simulink model "PID_C_R_Simulink_1_0_OLC"  (R2020a)
settings: Solver=FixedStepAuto  StartTime=0.0  StopTime=inf  RelTol=1e-3  EnableMultiTasking=on
libraries: arduinolib x8, simulink x2
Description:
  | __Simple PID driven robot
  | ___Open loop control
settings Model: SILPILModeSetting=veronly  ExtModeTrigDuration=2  Creator=Mohanad M.Marzouk  LastModifiedBy=Mohanad M.Marzouk
settings SolverCC: AutoInsertRateTranBlk=on
settings OptimizationCC: EnhancedBackFolding=on  PassReuseOutputArgsAs=Individual arguments  ZeroExternalMemoryAtStartup=off  ZeroInternalMemoryAtStartup=off  MaxStackSize=64  OptimizeBlockOrder=speed  DifferentSizesBufferReuse=on  OptimizationCustomize=off  EfficientTunableParamExpr=on
settings DebuggingCC: ParameterTunabilityLossMsg=error
settings HardwareCC: ProdBitPerInt=16  ProdBitPerPointer=16  ProdBitPerSizeT=16  ProdBitPerPtrDiffT=16  ProdLargestAtomicFloat=None  ProdWordSize=8  ProdHWDeviceType=Atmel->AVR
settings SFSimCC: MATLABDynamicMemAlloc=off
settings RTWCC: SystemTargetFile=ert.tlc  HardwareBoard=Arduino Mega 2560  TLCOptions=-aInlineSetEventsForThisBaseRateFcn=TLC_FALSE -aSuppressMultiTaskScheduler=TLC_FALSE -aRateBasedStepFcn=1  GenCodeOnly=on  TemplateMakefile=ert_default_tmf  Toolchain=Arduino AVR  BuildConfiguration=Faster Runs
settings CodeAppCC: ForceParamTrailComments=on  IgnoreCustomStorageClasses=off  OperatorAnnotations=on  SimulinkDataObjDesc=on  SFDataObjDesc=on  InsertBlockDesc=on
settings ERTTargetCC: SupportContinuousTime=on  SupportVariableSizeSignals=on  ExtModeStaticAllocSize=2048

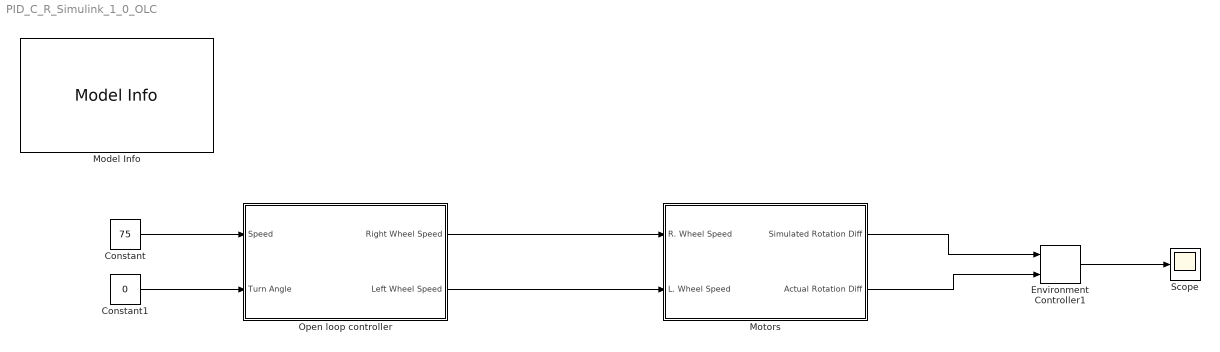
== system PID_C_R_Simulink_1_0_OLC ==
  Constant : Constant  Value=75
  Constant1 : Constant  Value=0
  Environment Controller1 : simulink/Signal Routing/Environment Controller
      settings: SourceProductBaseCode=SL
  Model Info : simulink/Model-Wide Utilities/Model Info  Frame=on  DisplayStringWithTags=|  HorizontalTextAlignment=Left  LeftAlignmentValue=0.02
      | Model Info
      | ---------------------------------------------
      | %<Created>
      | %<Creator>
      | %<ModelVersion>
      | %<ModelName>
      | %<Description>
      | %<LastModifiedBy>
      | %<LastModificationDate>
  Motors : Subsystem
  Open loop controller : Subsystem
  Scope : Scope
  wires:
  Environment Controller1/1 -> Scope/1
  Constant/1 -> Open loop controller/1(Speed)
  Constant1/1 -> Open loop controller/2(Turn Angle)
  Motors/1(Simulated Rotation Diff) -> Environment Controller1/1
  Motors/2(Actual Rotation Diff) -> Environment Controller1/2
  Open loop controller/1(Right Wheel Speed) -> Motors/1(R. Wheel Speed)
  Open loop controller/2(Left Wheel Speed) -> Motors/2(L. Wheel Speed)

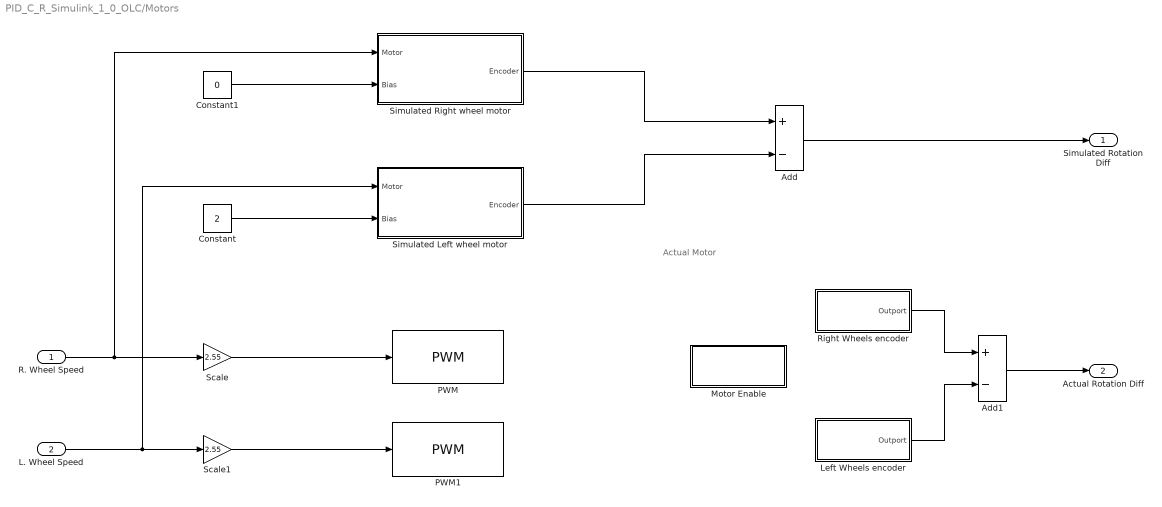
== system PID_C_R_Simulink_1_0_OLC/Motors ==
  note: Actual Motor
  R. Wheel Speed : Inport
  L. Wheel Speed : Inport  Port=2
  Add : Sum  Inputs=+-
  Add1 : Sum  Inputs=+-
  Constant : Constant  Value=2
  Constant1 : Constant  Value=0
  Left Wheels encoder : Subsystem
  Motor Enable : Subsystem
  PWM : arduinolib/PWM  pinNumber=10  frequencyType=Default  desiredFrequency=490.2  achievableFrequency=490.2
  PWM1 : arduinolib/PWM  pinNumber=11  frequencyType=Default  desiredFrequency=490.2  achievableFrequency=490.2
  Right Wheels encoder : Subsystem
  Scale : Gain  Gain=2.55
  Scale1 : Gain  Gain=2.55
  Simulated Left wheel motor : Subsystem
  Simulated Right wheel motor : Subsystem
  Simulated Rotation Diff : Outport
  Actual Rotation Diff : Outport  Port=2
  wires:
  Scale/1 -> PWM/1
  Scale1/1 -> PWM1/1
  L. Wheel Speed/1 -> Simulated Left wheel motor/1(Motor), Scale1/1
  R. Wheel Speed/1 -> Simulated Right wheel motor/1(Motor), Scale/1
  Constant/1 -> Simulated Left wheel motor/2(Bias)
  Constant1/1 -> Simulated Right wheel motor/2(Bias)
  Simulated Right wheel motor/1(Encoder) -> Add/1
  Simulated Left wheel motor/1(Encoder) -> Add/2
  Add/1 -> Simulated Rotation Diff/1
  Add1/1 -> Actual Rotation Diff/1
  Left Wheels encoder/1(Outport) -> Add1/2
  Right Wheels encoder/1(Outport) -> Add1/1

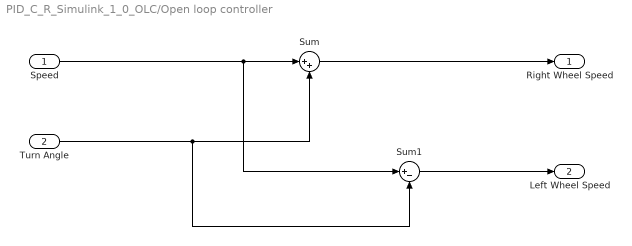
== system PID_C_R_Simulink_1_0_OLC/Open loop controller ==
  Speed : Inport
  Turn Angle : Inport  Port=2
  Sum : Sum  Inputs=|++
  Sum1 : Sum  Inputs=|+-
  Right Wheel Speed : Outport
  Left Wheel Speed : Outport  Port=2
  wires:
  Sum/1 -> Right Wheel Speed/1
  Sum1/1 -> Left Wheel Speed/1
  Turn Angle/1 -> Sum1/2, Sum/2
  Speed/1 -> Sum1/1, Sum/1

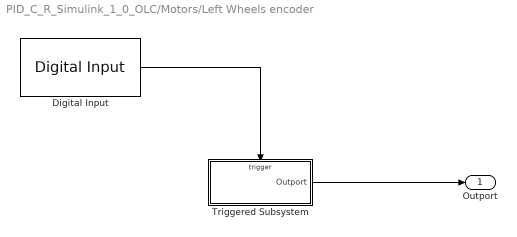
== system PID_C_R_Simulink_1_0_OLC/Motors/Left Wheels encoder ==
  Digital Input : arduinolib/Digital Input  pinNumber=9  Direction=input  SampleTime=0.001  blockPlatform=arduino
  Triggered Subsystem : Subsystem  TreatAsAtomicUnit=on
  Outport : Outport
  wires:
  Digital Input/1 -> Triggered Subsystem/Trigger
  Triggered Subsystem/1(Outport) -> Outport/1

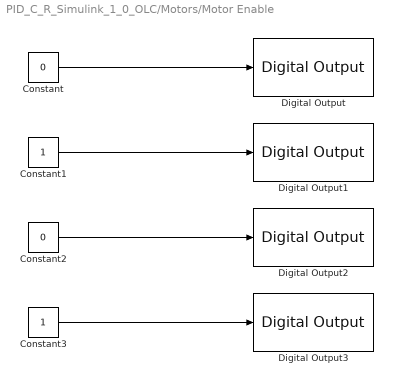
== system PID_C_R_Simulink_1_0_OLC/Motors/Motor Enable ==
  Constant : Constant  Value=0
  Constant1 : Constant
  Constant2 : Constant  Value=0
  Constant3 : Constant
  Digital Output : arduinolib/Digital Output  pinNumber=4  Direction=output  blockPlatform=arduino
  Digital Output1 : arduinolib/Digital Output  pinNumber=5  Direction=output  blockPlatform=arduino
  Digital Output2 : arduinolib/Digital Output  pinNumber=2  Direction=output  blockPlatform=arduino
  Digital Output3 : arduinolib/Digital Output  pinNumber=3  Direction=output  blockPlatform=arduino
  wires:
  Constant/1 -> Digital Output/1
  Constant1/1 -> Digital Output1/1
  Constant2/1 -> Digital Output2/1
  Constant3/1 -> Digital Output3/1

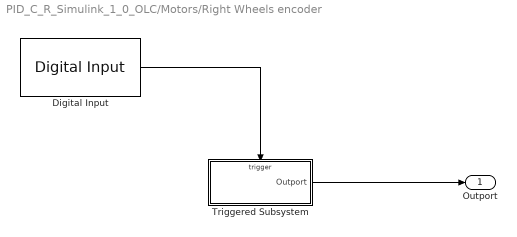
== system PID_C_R_Simulink_1_0_OLC/Motors/Right Wheels encoder ==
  Digital Input : arduinolib/Digital Input  pinNumber=8  Direction=input  SampleTime=0.001  blockPlatform=arduino
  Triggered Subsystem : Subsystem  TreatAsAtomicUnit=on
  Outport : Outport
  wires:
  Triggered Subsystem/1(Outport) -> Outport/1
  Digital Input/1 -> Triggered Subsystem/Trigger

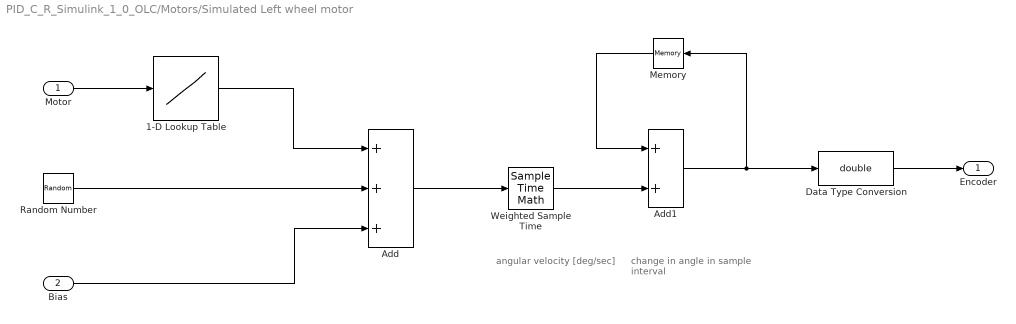
== system PID_C_R_Simulink_1_0_OLC/Motors/Simulated Left wheel motor ==
  note: change in angle
      | in sample interval
  note: angular velocity
      | [deg/sec]
  Motor : Inport
  Bias : Inport  Port=2
  1-D Lookup Table : Lookup_n-D  NumberOfTableDimensions=1  BreakpointsForDimension1=[-100,0,100]  Table=[-360,0,360]  ExtrapMethod=Clip  UseLastTableValue=on  InternalRulePriority=Speed  RndMeth=Simplest  InputSameDT=on
  Add : Sum  Inputs=+++
  Add1 : Sum
  Data Type Conversion : DataTypeConversion  OutDataTypeStr=double  LockScale=on
  Memory : Memory
  Random Number : RandomNumber  Variance=5  Seed=randi(1000)  SampleTime=0.1
  Weighted Sample Time : SampleTimeMath  TsampMathOp=*
  Encoder : Outport
  wires:
  Memory/1 -> Add1/1
  Add1/1 -> Data Type Conversion/1, Memory/1
  Data Type Conversion/1 -> Encoder/1
  Weighted Sample Time/1 -> Add1/2
  Add/1 -> Weighted Sample Time/1
  Bias/1 -> Add/3
  Random Number/1 -> Add/2
  1-D Lookup Table/1 -> Add/1
  Motor/1 -> 1-D Lookup Table/1

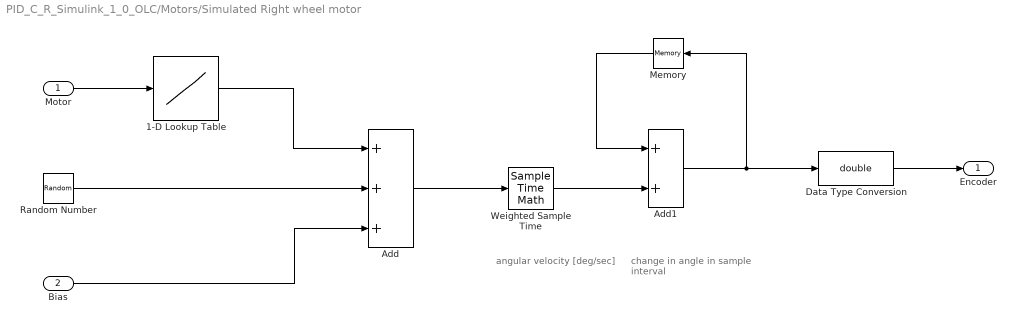
== system PID_C_R_Simulink_1_0_OLC/Motors/Simulated Right wheel motor ==
  note: angular velocity
      | [deg/sec]
  note: change in angle
      | in sample interval
  Motor : Inport
  Bias : Inport  Port=2
  1-D Lookup Table : Lookup_n-D  NumberOfTableDimensions=1  BreakpointsForDimension1=[-100,0,100]  Table=[-360,0,360]  ExtrapMethod=Clip  UseLastTableValue=on  InternalRulePriority=Speed  RndMeth=Simplest  InputSameDT=on
  Add : Sum  Inputs=+++
  Add1 : Sum
  Data Type Conversion : DataTypeConversion  OutDataTypeStr=double  LockScale=on
  Memory : Memory
  Random Number : RandomNumber  Variance=5  Seed=randi(1000)  SampleTime=0.1
  Weighted Sample Time : SampleTimeMath  TsampMathOp=*
  Encoder : Outport
  wires:
  Motor/1 -> 1-D Lookup Table/1
  1-D Lookup Table/1 -> Add/1
  Random Number/1 -> Add/2
  Bias/1 -> Add/3
  Add/1 -> Weighted Sample Time/1
  Weighted Sample Time/1 -> Add1/2
  Data Type Conversion/1 -> Encoder/1
  Add1/1 -> Memory/1, Data Type Conversion/1
  Memory/1 -> Add1/1

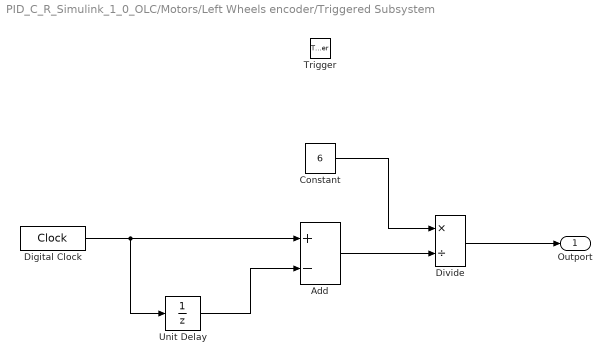
== system PID_C_R_Simulink_1_0_OLC/Motors/Left Wheels encoder/Triggered Subsystem ==
  Trigger : TriggerPort  VariantControl=Variant
  Add : Sum  Inputs=+-
  Constant : Constant  Value=6
  Digital Clock : DigitalClock  SampleTime=-1
  Divide : Product  Inputs=*/
  Unit Delay : UnitDelay  SampleTime=-1  HasFrameUpgradeWarning=on
  Outport : Outport
  wires:
  Divide/1 -> Outport/1
  Add/1 -> Divide/2
  Constant/1 -> Divide/1
  Unit Delay/1 -> Add/2
  Digital Clock/1 -> Add/1, Unit Delay/1

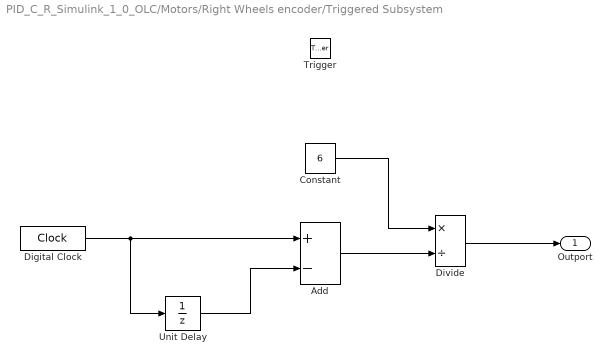
== system PID_C_R_Simulink_1_0_OLC/Motors/Right Wheels encoder/Triggered Subsystem ==
  Trigger : TriggerPort  VariantControl=Variant
  Add : Sum  Inputs=+-
  Constant : Constant  Value=6
  Digital Clock : DigitalClock  SampleTime=-1
  Divide : Product  Inputs=*/
  Unit Delay : UnitDelay  SampleTime=-1  HasFrameUpgradeWarning=on
  Outport : Outport
  wires:
  Digital Clock/1 -> Unit Delay/1, Add/1
  Unit Delay/1 -> Add/2
  Constant/1 -> Divide/1
  Add/1 -> Divide/2
  Divide/1 -> Outport/1
